simulink model "traj_tracking"  (R2022a)
settings: Solver=VariableStepAuto  StartTime=0.0  StopTime=20.0  FixedStep=0.01  MaxStep=0.01  RelTol=1e-3
values from neighbouring files (symbols this model uses):
  Kd_b = diag(getBlockParam(st, 'Kd_b').Gain.Value)    [ctrl_synth.m]
  Kd_m = diag(getBlockParam(st, 'Kd_m').Gain.Value)    [ctrl_synth.m]
  Kp_b = diag(getBlockParam(st, 'Kp_b').Gain.Value)    [ctrl_synth.m]
  Kp_m = diag(getBlockParam(st, 'Kp_m').Gain.Value)    [ctrl_synth.m]
  n = robot.n_links_joints    [CIM_test.m]    (also in ctrl_synth.m = sc.NumActiveJoints; dh_test.m = 2; dh_test_2.m = size(dhparams, 1); ee_dyn_check.m = sr6.NumActiveJoints)
  sc = SpaceRobot    [model_test.m]    (also in test.m = SpaceRobot('SC_2DoF.urdf'))
undefined symbols (not defined in the file or in its folder): dA
libraries: dspmathops x1
settings Model: Creator=charl  LastModifiedBy=charl

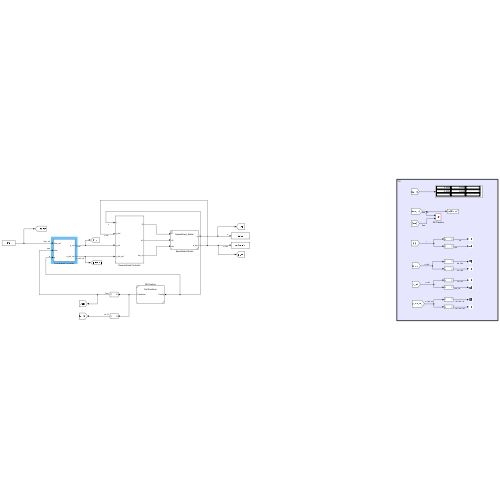
[thumbnail: Simulink's stored preview of the top-level diagram]
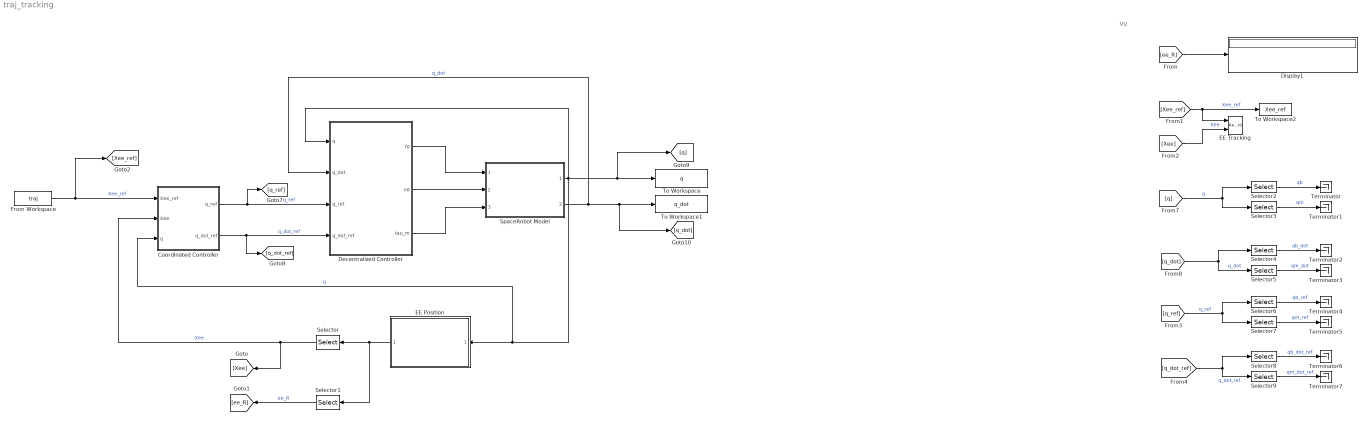
== system traj_tracking ==
  note: Viz
  Coordinated Controller : Subsystem  mask(Coordinated Controller){spaceRobot=sc, dA=dA, Gb=0, Gm=0}
      mask prompts: spaceRobot "Space Robot:"
      mask help: Computes the joints angle and base coordinated to follow the trajectory
  Decentralized Controller : Subsystem  mask(Decentralized Controller){Kp_b=Kp_b, Kd_b=Kd_b, Kp_m=Kp_m, Kd_m=Kd_m}
      mask prompts: Kp_b "Kp:"; Kd_b "Kd:"; Kp_m "Kp:"; Kd_m "Kd:"
      mask help:
      | Inner Loop control of SpaceRobot.
      | Input gains as vector that will be used as diagonal of gain matrix.
      | n: # DoF of manipulator
      |
      | Base:
      | - Kp (6x1)
      | - Kd (6x1)
      |
      | Manipulator
      | - Kp (nx1)
      | - Kd (nx1)
      mask DialogControl ParameterGroupVar Prompt: Base
      mask DialogControl ParameterGroupVar_copy Prompt: Manipulator
  Display1 : Display
  EE Position : Subsystem  ReferencedSubsystem=GetTransform  spaceRobot=sc  sourceLink=endeffector  targetLink=inertial  SimulateUsing=Interpreted execution
  EE Tracking : Record  FileSettingsInternal="{\"entries\":[{\"content\":{\"excelSettings\":{\"content\":{},\"type\":\"Streamout.ExcelSettings\"}},\"type\":\"Streamout.FileSettingStorage\",\"uuid\":\"66fa77df-fe9a-4656-9320-a3be1868e35e\"}],\"packageUris\":[\"http://schema.mathworks.com/mf0/streamout_blocks/R2020a\"],\"version\":\"1.0\"}"  Layout=[1 1]  SignalsInternal="{\"entries\":[{\"content\":{\"signals\":[{\"content\":{\"blockPath\":[\"traj_tracking/EE Tracking\"],\"channel\":[],\"dimensions\":[3,1],\"domain\":\"traj_tracking/EE Tracking\",\"hasChildren\":true,\"lineColor\":\"#4dbeee\",\"plots\":[],\"port\":1,\"sid\":[\"\"],\"signalID\":17598,\"signalName\":\"Xee_ref\"},\"type\":\"RecordBlkView.Signal\",\"uuid\":\"6c242f46-2f15-4d93-b2f4-d6e6f6733dfe\"},{\"content\":{\"blockPath\":[\"traj_tracking/EE Tracking\"],\"channel\":[1,1],\"dimensions\":[3,1],\"domain\":\"traj_tracking/EE Tracking\",\"lineColor\":\"#fe330a\",\"parentID\":17598,\"plots\":[1],\"port\":1,\"sid\":[\"\"],\"signalID\":17599,\"signalName\":\"Xee_ref\"},\"type\":\"RecordBlkView.Signal\",\"uuid\":\"a9df4cb9-e3b2-405d-9232-f6c036fa5177\"},{\"content\":{\"blockPath\":[\"traj_tracking/EE Tracking\"],\"channel\":[],\"dimensions\":[3,1],\"domain\":\"traj_tracking/EE Tracking\",\"hasChildren\":true,\"lineColor\":\"#139fff\",\"plots\":[],\"port\":2,\"sid\":[\"\"],\"signalID\":17603,\"signalName\":\"Xee\"},\"type\":\"RecordBlkView.Signal\",\"uuid\":\"a67fe54e-95a0-415c-b922-7742b02257b4\"},{\"content\":{\"blockPath\":[\"traj_tracking/EE Tracking\"],\"channel\":[1,1],\"dimensions\":[3,1],\"domain\":\"traj_tracking/EE Tracking\",\"lineColor\":\"#4dbeee\",\"parentID\":17603,\"plots\":[1],\"port\":2,\"sid\":[\"\"],\"signalID\":17604,\"signalName\":\"Xee\"},\"type\":\"RecordBlkView.Signal\",\"uuid\":\"03c16471-32f0-4102-b1cc-17d321a16556\"},{\"content\":{\"blockPath\":[\"traj_tracking/EE Tracking\"],\"channel\":[2,1],\"dimensions\":[3,1],\"domain\":\"traj_tracking/EE Tracking\",\"lineColor\":\"#fe330a\",\"parentID\":17598,\"plots\":[1],\"port\":1,\"sid\":[\"\"],\"signalID\":17656,\"signalName\":\"Xee_ref\"},\"type\":\"RecordBlkView.Signal\",\"uuid\":\"1c37c4c2-48fd-419d-af06-1d771213a662\"},{\"content\":{\"blockPath\":[\"traj_tracking/EE Tracking\"],\"channel\":[3,1],\"dimensions\":[3,1],\"domain\":\"traj_tracking/EE Tracking\",\"lineColor\":\"#a2142f\",\"parentID\":17598,\"plots\":[],\"port\":1,\"sid\":[\"\"],\"signalID\":17657,\"signalName\":\"Xee_ref\"},\"type\":\"RecordBlkView.Signal\",\"uuid\":\"19202850-31de-429d-a5ec-31ed1f91d639\"},{\"content\":{\"blockPath\":[\"traj_tracking/EE Tracking\"],\"channel\":[2,1],\"dimensions\":[3,1],\"domain\":\"traj_tracking/EE Tracking\",\"lineColor\":\"#4dbeee\",\"parentID\":17603,\"plots\":[1],\"port\":2,\"sid\":[\"\"],\"signalID\":17658,\"signalName\":\"Xee\"},\"type\":\"RecordBlkView.Signal\",\"uuid\":\"46bd9c3c-a809-4561-b9e7-569eea1bc161\"},{\"content\":{\"blockPath\":[\"traj_tracking/EE Tracking\"],\"channel\":[3,1],\"dimensions\":[3,1],\"domain\":\"traj_tracking/EE Tracking\",\"lineColor\":\"#ff6929\",\"parentID\":17603,\"plots\":[],\"port\":2,\"sid\":[\"\"],\"signalID\":17659,\"signalName\":\"Xee\"},\"type\":\"RecordBlkView.Signal\",\"uuid\":\"6c26f334-ea13-4214-8424-f96231f93691\"}]},\"type\":\"RecordBlkView.InputSignals\",\"uuid\":\"344cecc8-bf5c-4716-aea7-c87ba6653e99\"}],\"packageUris\":[\"http://schema.mathworks.com/mf0/streamout_blocks/R2020a\"],\"version\":\"1.0\"}"  VisualizationBindings="{\"xyplotplugin\":{\"info\":[{\"series\":[{\"bindingParametersList\":[{\"parameter\":\"Y-Axis\",\"signalID\":17658,\"signalName\":\"Xee(2,1)\"},{\"parameter\":\"X-Axis\",\"signalID\":17604,\"signalName\":\"Xee(1,1)\"}],\"seriesID\":9779},{\"bindingParametersList\":[{\"parameter\":\"X-Axis\",\"signalID\":17599,\"signalName\":\"Xee_ref(1,1)\"},{\"parameter\":\"Y-Axis\",\"signalID\":17656,\"signalName\":\"Xee_ref(2,1)\"}],\"seriesID\":293}],\"subplotID\":1}]}}"  CompatibilityTag=XY
  From Workspace : FromWorkspace  VariableName=traj
  Selector : Selector  NumberOfDimensions=2  InputPortWidth=[4 4]  IndexOptions=Index vector (dialog),Index vector (dialog)  Indices=[1:3],4  OutputSizes=1,1
  Selector1 : Selector  NumberOfDimensions=2  InputPortWidth=[4 4]  IndexOptions=Index vector (dialog),Index vector (dialog)  Indices=[1:3],[1:3]  OutputSizes=1,1
  Selector{2,4,6,8} (4 alike) : Selector  IndexOptions=Index vector (dialog)  Indices=[1:6]  OutputSizes=1
  Selector{3,5,7,9} (4 alike) : Selector  IndexOptions=Index vector (dialog)  Indices=[7:6+n]  OutputSizes=1
  SpaceRobot Model : Subsystem  ReferencedSubsystem=SpaceRobot_Model  spaceRobot=sc
  Terminator{,1..7} (8 alike) : Terminator
  To Workspace : ToWorkspace  VariableName=q  SaveFormat=Timeseries  SampleTime=-1
  To Workspace1 : ToWorkspace  VariableName=q_dot  SaveFormat=Timeseries  SampleTime=-1
  To Workspace2 : ToWorkspace  VariableName=Xee_ref  SaveFormat=Timeseries  SampleTime=-1
  wires:
  From Workspace/1 -> Coordinated Controller/1(Xee_ref), [Xee_ref]  "Xee_ref"
  EE Position/1 -> Selector1/1, Selector/1
  Selector/1 -> Coordinated Controller/2(Xee), [Xee]  "Xee"
  SpaceRobot Model/2 -> Decentralized Controller/2(q_dot), [q_dot], To Workspace1/1  "q_dot"
  SpaceRobot Model/1 -> Decentralized Controller/1(q), [q], To Workspace/1, Coordinated Controller/3(q), EE Position/1  "q"
  [ee_R] -> Display1/1
  Selector1/1 -> [ee_R]  "ee_R"
  [Xee_ref] -> To Workspace2/1, EE Tracking/1  "Xee_ref"
  [Xee] -> EE Tracking/2  "Xee"
  Decentralized Controller/1(f0) -> SpaceRobot Model/1
  Decentralized Controller/2(n0) -> SpaceRobot Model/2
  Decentralized Controller/3(tau_m) -> SpaceRobot Model/3
  Coordinated Controller/1(q_ref) -> [q_ref], Decentralized Controller/3(q_ref)  "q_ref"
  Coordinated Controller/2(q_dot_ref) -> [q_dot_ref], Decentralized Controller/4(q_dot_ref)  "q_dot_ref"
  [q] -> Selector3/1, Selector2/1  "q"
  Selector4/1 -> Terminator2/1  "qb_dot"
  Selector2/1 -> Terminator/1  "qb"
  [q_dot] -> Selector4/1, Selector5/1  "q_dot"
  Selector5/1 -> Terminator3/1  "qm_dot"
  Selector6/1 -> Terminator4/1  "qb_ref"
  [q_ref] -> Selector7/1, Selector6/1  "q_ref"
  Selector8/1 -> Terminator6/1  "qb_dot_ref"
  [q_dot_ref] -> Selector9/1, Selector8/1  "q_dot_ref"
  Selector9/1 -> Terminator7/1  "qm_dot_ref"
  Selector3/1 -> Terminator1/1  "qm"
  Selector7/1 -> Terminator5/1  "qm_ref"

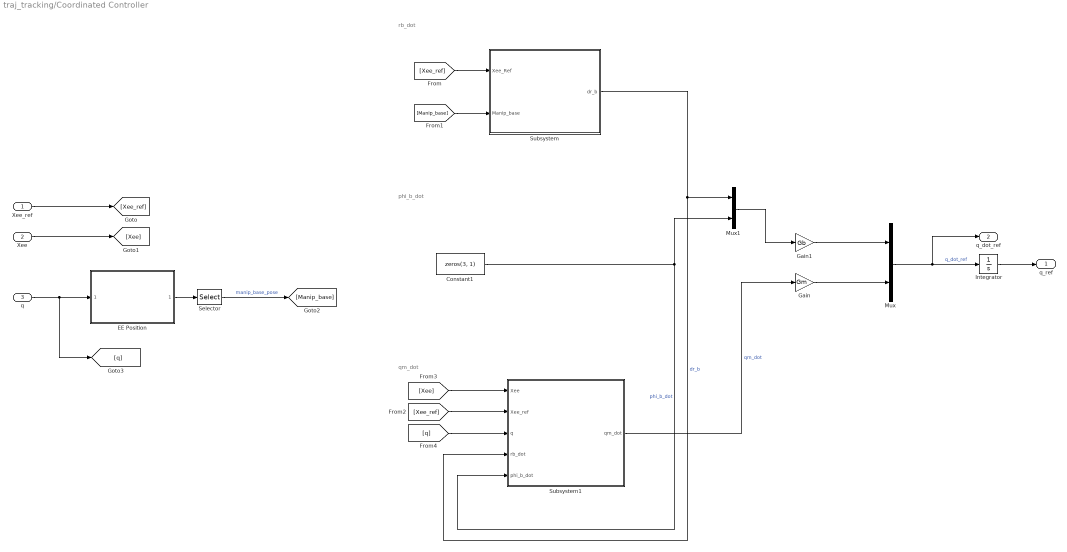
== system traj_tracking/Coordinated Controller ==
  note: rb_dot
  note: phi_b_dot
  note: qm_dot
  Xee_ref : Inport
  Xee : Inport  Port=2
  q : Inport  Port=3
  Constant1 : Constant  Value=zeros(3, 1)
  EE Position : Subsystem  ReferencedSubsystem=GetTransform  spaceRobot=spaceRobot  sourceLink=Link1  targetLink=inertial  SimulateUsing=Interpreted execution
  Gain : Gain  Gain=Gm
  Gain1 : Gain  Gain=Gb
  Integrator : Integrator  InitialCondition=sc.q
  Mux : Mux  Inputs=2
  Mux1 : Mux  Inputs=2
  Selector : Selector  NumberOfDimensions=2  InputPortWidth=[4 4]  IndexOptions=Index vector (dialog),Index vector (dialog)  Indices=[1:3],4  OutputSizes=1,1
  Subsystem : Subsystem
  Subsystem1 : Subsystem
  q_ref : Outport
  q_dot_ref : Outport  Port=2
  wires:
  q/1 -> [q], EE Position/1
  EE Position/1 -> Selector/1
  Selector/1 -> [Manip_base]  "manip_base_pose"
  Constant1/1 -> Mux1/2, Subsystem1/5(phi_b_dot)  "phi_b_dot"
  Mux/1 -> q_dot_ref/1, Integrator/1  "q_dot_ref"
  Integrator/1 -> q_ref/1
  Subsystem1/1(qm_dot) -> Gain/1  "qm_dot"
  Xee_ref/1 -> [Xee_ref]
  Subsystem/1(dr_b) -> Subsystem1/4(rb_dot), Mux1/1  "dr_b"
  Xee/1 -> [Xee]
  [Xee_ref] -> Subsystem/1(Xee_Ref)
  [Manip_base] -> Subsystem/2(Manip_base)
  [Xee_ref] -> Subsystem1/2(Xee_ref)
  [Xee] -> Subsystem1/1(Xee)
  [q] -> Subsystem1/3(q)
  Gain1/1 -> Mux/1
  Gain/1 -> Mux/2
  Mux1/1 -> Gain1/1

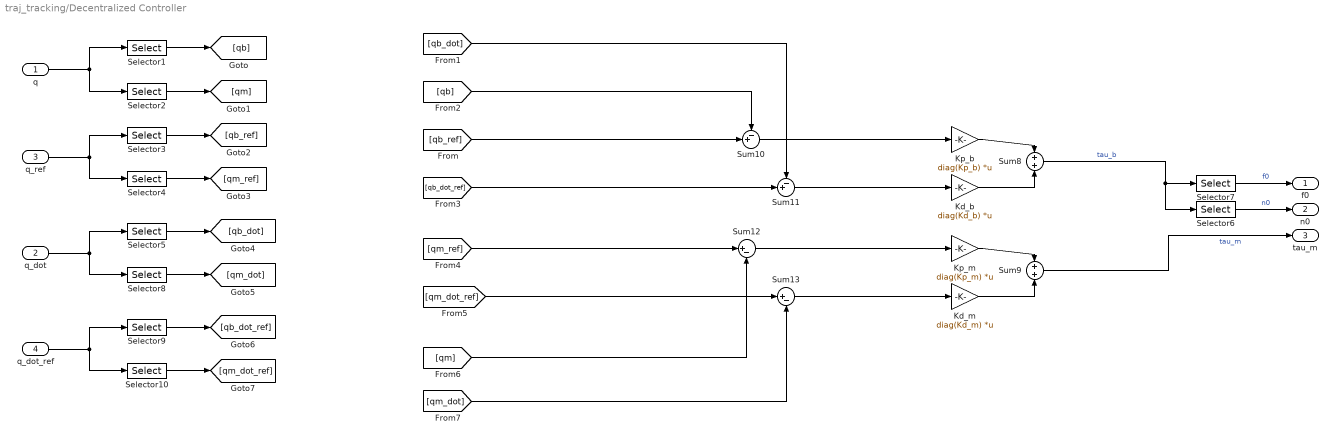
== system traj_tracking/Decentralized Controller ==
  q : Inport
  q_dot : Inport  Port=2
  q_ref : Inport  Port=3
  q_dot_ref : Inport  Port=4
  Kd_b : Gain  Gain=diag(Kd_b)  Multiplication=Matrix(K*u)
  Kd_m : Gain  Gain=diag(Kd_m)  Multiplication=Matrix(K*u)
  Kp_b : Gain  Gain=diag(Kp_b)  Multiplication=Matrix(K*u)
  Kp_m : Gain  Gain=diag(Kp_m)  Multiplication=Matrix(K*u)
  Selector{1,3,5,9} (4 alike) : Selector  IndexOptions=Index vector (dialog)  Indices=[1:6]  OutputSizes=1
  Selector{2,4,8,10} (4 alike) : Selector  IndexOptions=Index vector (dialog)  Indices=[7:6+n]  OutputSizes=1
  Selector6 : Selector  IndexOptions=Index vector (dialog)  Indices=[4:6]  OutputSizes=1
  Selector7 : Selector  IndexOptions=Index vector (dialog)  Indices=[1:3]  OutputSizes=1
  Sum10 : Sum  Inputs=-+|
  Sum11 : Sum  Inputs=-+|
  Sum12 : Sum  Inputs=|+-
  Sum13 : Sum  Inputs=|+-
  Sum8 : Sum  Inputs=+|+
  Sum9 : Sum  Inputs=+|+
  f0 : Outport
  n0 : Outport  Port=2
  tau_m : Outport  Port=3
  wires:
  Sum8/1 -> Selector6/1, Selector7/1  "tau_b"
  Kd_b/1 -> Sum8/2
  [qb] -> Sum10/1
  Sum10/1 -> Kp_b/1
  [qm_ref] -> Sum12/1
  Sum12/1 -> Kp_m/1
  Sum11/1 -> Kd_b/1
  [qm_dot_ref] -> Sum13/1
  Sum9/1 -> tau_m/1  "tau_m"
  Kd_m/1 -> Sum9/2
  Kp_b/1 -> Sum8/1
  Sum13/1 -> Kd_m/1
  Kp_m/1 -> Sum9/1
  [qm_dot] -> Sum13/2
  [qb_dot] -> Sum11/1
  [qb_dot_ref] -> Sum11/2
  Selector7/1 -> f0/1  "f0"
  Selector6/1 -> n0/1  "n0"
  [qb_ref] -> Sum10/2
  [qm] -> Sum12/2
  q/1 -> Selector2/1, Selector1/1
  Selector1/1 -> [qb]
  Selector2/1 -> [qm]
  Selector3/1 -> [qb_ref]
  Selector4/1 -> [qm_ref]
  q_ref/1 -> Selector4/1, Selector3/1
  Selector8/1 -> [qm_dot]
  Selector5/1 -> [qb_dot]
  q_dot/1 -> Selector8/1, Selector5/1
  Selector10/1 -> [qm_dot_ref]
  Selector9/1 -> [qb_dot_ref]
  q_dot_ref/1 -> Selector10/1, Selector9/1

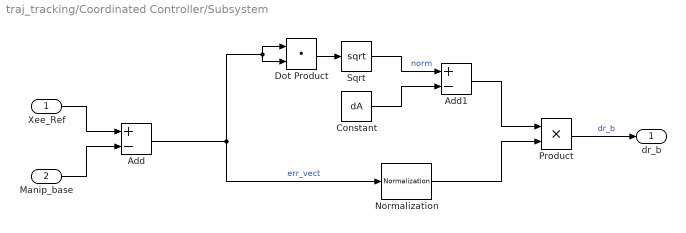
== system traj_tracking/Coordinated Controller/Subsystem ==
  Xee_Ref : Inport
  Manip_base : Inport  Port=2
  Add : Sum  Inputs=+-
  Add1 : Sum  Inputs=+-
  Constant : Constant  Value=dA
  Dot Product : DotProduct  OutDataTypeStr=Inherit: Inherit via internal rule
  Normalization : dspmathops/Normalization  NormType=2-norm  Bias=1e-10  NormOver=Each column  Dimension=1  roundingMode=Floor  overflowMode=off  accumDataTypeStr=Inherit: Same as product output  accumLastDataTypeStr=Inherit: Same as product output  outputDataTypeStr=Inherit: Same as product output  outputMin=[]  outputMax=[]  outputLastDataTypeStr=Inherit: Same as product output
  Product : Product
  Sqrt : Sqrt
  dr_b : Outport
  wires:
  Manip_base/1 -> Add/2
  Dot Product/1 -> Sqrt/1
  Product/1 -> dr_b/1  "dr_b"
  Constant/1 -> Add1/2
  Normalization/1 -> Product/2
  Xee_Ref/1 -> Add/1
  Add1/1 -> Product/1
  Sqrt/1 -> Add1/1  "norm"
  Add/1 -> Dot Product/1, Dot Product/2, Normalization/1  "err_vect"

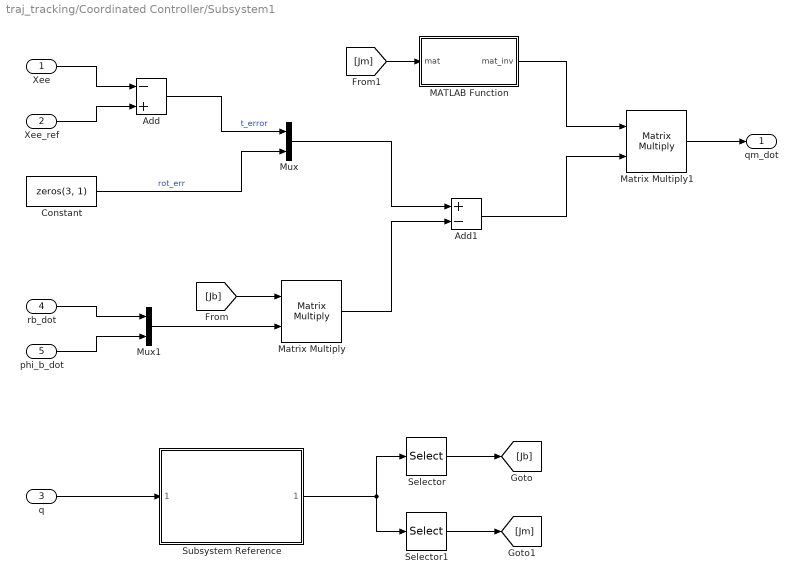
== system traj_tracking/Coordinated Controller/Subsystem1 ==
  Xee : Inport
  Xee_ref : Inport  Port=2
  q : Inport  Port=3
  rb_dot : Inport  Port=4
  phi_b_dot : Inport  Port=5
  Add : Sum  Inputs=-+
  Add1 : Sum  Inputs=+-
  Constant : Constant  Value=zeros(3, 1)
  MATLAB Function : MATLAB Function  TreatAsAtomicUnit=on
  Matrix Multiply : Product  Multiplication=Matrix(*)
  Matrix Multiply1 : Product  Multiplication=Matrix(*)
  Mux : Mux  Inputs=2
  Mux1 : Mux  Inputs=2
  Selector : Selector  NumberOfDimensions=2  InputPortWidth=3  IndexOptions=Index vector (dialog),Index vector (dialog)  Indices=[1:6],[1:6]  OutputSizes=1,1
  Selector1 : Selector  NumberOfDimensions=2  InputPortWidth=3  IndexOptions=Index vector (dialog),Index vector (dialog)  Indices=[1:6],[7:6+n]  OutputSizes=1,1
  Subsystem Reference : Subsystem  ReferencedSubsystem=GetJacobian  spaceRobot=spaceRobot  sourceLink=endeffector  SimulateUsing=Interpreted execution
  qm_dot : Outport
  wires:
  Xee_ref/1 -> Add/2
  q/1 -> Subsystem Reference/1
  Xee/1 -> Add/1
  phi_b_dot/1 -> Mux1/2
  Selector/1 -> [Jb]
  Add1/1 -> Matrix Multiply1/2
  Constant/1 -> Mux/2  "rot_err"
  [Jm] -> MATLAB Function/1(mat)
  Matrix Multiply/1 -> Add1/2
  Add/1 -> Mux/1  "t_error"
  Mux1/1 -> Matrix Multiply/2
  Selector1/1 -> [Jm]
  MATLAB Function/1(mat_inv) -> Matrix Multiply1/1
  Matrix Multiply1/1 -> qm_dot/1
  Mux/1 -> Add1/1
  Subsystem Reference/1 -> Selector1/1, Selector/1
  [Jb] -> Matrix Multiply/1
  rb_dot/1 -> Mux1/1

== matlab function traj_tracking/Coordinated Controller/Subsystem1/MATLAB Function ==
  data: mat input; mat_inv output
function mat_inv = fcn(mat)

mat_inv = pinv(mat);
